simulink model "bicycle_car_model"  (R2019b)
settings: Solver=ode45  StartTime=0.0  StopTime=tf  MaxStep=0.01  RelTol=1e-3
undefined symbols (not defined in the file): a, accel_noise, accel_ts, b, Cf, Cr_MR, Cr_R, d0, gyro_noise, gyro_ts, initial, Jy, Ku_MR, Ku_R, m, mag_noise, mag_ts, mu, Nf, Nr, sf, sr, ti, U
libraries: simulink x5
settings Model: Creator=lclemen  LastModifiedBy=lclemen

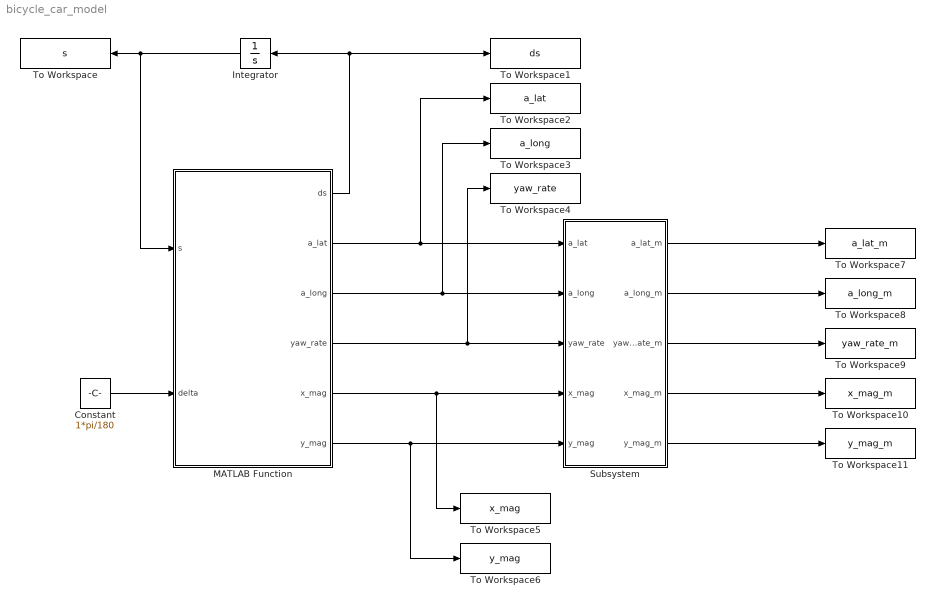
== system bicycle_car_model ==
  Constant : Constant  Value=1*pi/180
  Integrator : Integrator  InitialCondition=initial
  MATLAB Function : MATLAB Function  TreatAsAtomicUnit=on
  Subsystem : Subsystem
  To Workspace : ToWorkspace  VariableName=s  SampleTime=-1
      settings: Save2DSignal=2-D array (concatenate along first dimension)
  To Workspace1 : ToWorkspace  VariableName=ds  SampleTime=-1
      settings: Save2DSignal=2-D array (concatenate along first dimension)
  To Workspace10 : ToWorkspace  VariableName=x_mag_m  SampleTime=-1
      settings: Save2DSignal=2-D array (concatenate along first dimension)
  To Workspace11 : ToWorkspace  VariableName=y_mag_m  SampleTime=-1
      settings: Save2DSignal=2-D array (concatenate along first dimension)
  To Workspace2 : ToWorkspace  VariableName=a_lat  SampleTime=-1
      settings: Save2DSignal=2-D array (concatenate along first dimension)
  To Workspace3 : ToWorkspace  VariableName=a_long  SampleTime=-1
      settings: Save2DSignal=2-D array (concatenate along first dimension)
  To Workspace4 : ToWorkspace  VariableName=yaw_rate  SampleTime=-1
      settings: Save2DSignal=2-D array (concatenate along first dimension)
  To Workspace5 : ToWorkspace  VariableName=x_mag  SampleTime=-1
      settings: Save2DSignal=2-D array (concatenate along first dimension)
  To Workspace6 : ToWorkspace  VariableName=y_mag  SampleTime=-1
      settings: Save2DSignal=2-D array (concatenate along first dimension)
  To Workspace7 : ToWorkspace  VariableName=a_lat_m  SampleTime=-1
      settings: Save2DSignal=2-D array (concatenate along first dimension)
  To Workspace8 : ToWorkspace  VariableName=a_long_m  SampleTime=-1
      settings: Save2DSignal=2-D array (concatenate along first dimension)
  To Workspace9 : ToWorkspace  VariableName=yaw_rate_m  SampleTime=-1
      settings: Save2DSignal=2-D array (concatenate along first dimension)
  wires:
  MATLAB Function/2(a_lat) -> Subsystem/1(a_lat), To Workspace2/1
  MATLAB Function/1(ds) -> Integrator/1, To Workspace1/1
  Integrator/1 -> To Workspace/1, MATLAB Function/1(s)
  Constant/1 -> MATLAB Function/2(delta)
  MATLAB Function/3(a_long) -> Subsystem/2(a_long), To Workspace3/1
  MATLAB Function/4(yaw_rate) -> Subsystem/3(yaw_rate), To Workspace4/1
  MATLAB Function/6(y_mag) -> To Workspace6/1, Subsystem/5(y_mag)
  MATLAB Function/5(x_mag) -> To Workspace5/1, Subsystem/4(x_mag)
  Subsystem/1(a_lat_m) -> To Workspace7/1
  Subsystem/2(a_long_m) -> To Workspace8/1
  Subsystem/3(yaw_rate_m) -> To Workspace9/1
  Subsystem/4(x_mag_m) -> To Workspace10/1
  Subsystem/5(y_mag_m) -> To Workspace11/1

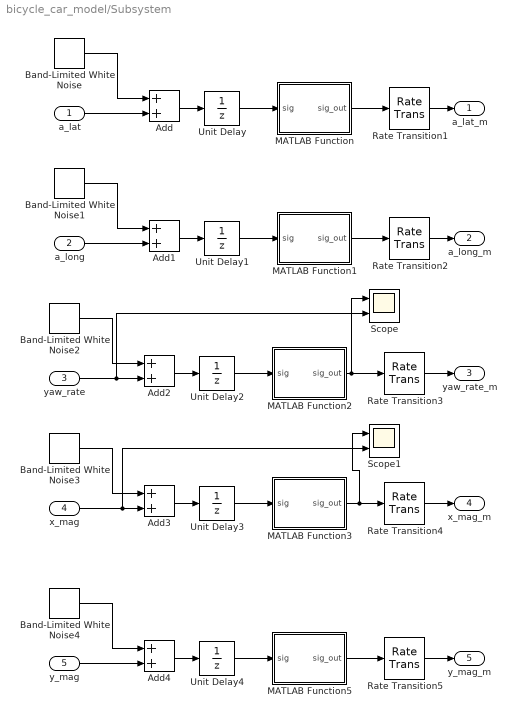
== system bicycle_car_model/Subsystem ==
  a_lat : Inport
  a_long : Inport  Port=2
  yaw_rate : Inport  Port=3
  x_mag : Inport  Port=4
  y_mag : Inport  Port=5
  Add{,1..4} (5 alike) : Sum
  Band-Limited White Noise : simulink/Sources/Band-Limited White Noise  Cov=[accel_noise]  Ts=0.001  seed=[23341]
  Band-Limited White Noise1 : simulink/Sources/Band-Limited White Noise  Cov=[accel_noise]  Ts=0.001  seed=[23341]
  Band-Limited White Noise2 : simulink/Sources/Band-Limited White Noise  Cov=[gyro_noise]  Ts=0.001  seed=[23341]
  Band-Limited White Noise3 : simulink/Sources/Band-Limited White Noise  Cov=[mag_noise]  Ts=0.001  seed=[23341]
  Band-Limited White Noise4 : simulink/Sources/Band-Limited White Noise  Cov=[accel_noise]  Ts=0.001  seed=[23341]
  MATLAB Function : MATLAB Function  TreatAsAtomicUnit=on
  MATLAB Function1 : MATLAB Function  TreatAsAtomicUnit=on
  MATLAB Function2 : MATLAB Function  TreatAsAtomicUnit=on
  MATLAB Function3 : MATLAB Function  TreatAsAtomicUnit=on
  MATLAB Function5 : MATLAB Function  TreatAsAtomicUnit=on
  Rate Transition{1..5} (5 alike) : RateTransition
  Scope : Scope  NumInputPorts=2
  Scope1 : Scope  NumInputPorts=2
  Unit Delay : UnitDelay  SampleTime=accel_ts  HasFrameUpgradeWarning=on
  Unit Delay1 : UnitDelay  SampleTime=accel_ts  HasFrameUpgradeWarning=on
  Unit Delay2 : UnitDelay  SampleTime=gyro_ts  HasFrameUpgradeWarning=on
  Unit Delay3 : UnitDelay  SampleTime=mag_ts  HasFrameUpgradeWarning=on
  Unit Delay4 : UnitDelay  SampleTime=accel_ts  HasFrameUpgradeWarning=on
  a_lat_m : Outport
  a_long_m : Outport  Port=2
  yaw_rate_m : Outport  Port=3
  x_mag_m : Outport  Port=4
  y_mag_m : Outport  Port=5
  wires:
  Band-Limited White Noise/1 -> Add/1
  a_lat/1 -> Add/2
  Add/1 -> Unit Delay/1
  Rate Transition1/1 -> a_lat_m/1
  Unit Delay/1 -> MATLAB Function/1(sig)
  MATLAB Function/1(sig_out) -> Rate Transition1/1
  Band-Limited White Noise1/1 -> Add1/1
  MATLAB Function1/1(sig_out) -> Rate Transition2/1
  Add1/1 -> Unit Delay1/1
  a_long/1 -> Add1/2
  Unit Delay1/1 -> MATLAB Function1/1(sig)
  Rate Transition2/1 -> a_long_m/1
  MATLAB Function2/1(sig_out) -> Scope/1, Rate Transition3/1
  Add2/1 -> Unit Delay2/1
  yaw_rate/1 -> Scope/2, Add2/2
  Unit Delay2/1 -> MATLAB Function2/1(sig)
  Band-Limited White Noise2/1 -> Add2/1
  Rate Transition3/1 -> yaw_rate_m/1
  MATLAB Function3/1(sig_out) -> Scope1/1, Rate Transition4/1
  Add3/1 -> Unit Delay3/1
  x_mag/1 -> Scope1/2, Add3/2
  Unit Delay3/1 -> MATLAB Function3/1(sig)
  Band-Limited White Noise3/1 -> Add3/1
  Rate Transition4/1 -> x_mag_m/1
  MATLAB Function5/1(sig_out) -> Rate Transition5/1
  Add4/1 -> Unit Delay4/1
  y_mag/1 -> Add4/2
  Unit Delay4/1 -> MATLAB Function5/1(sig)
  Band-Limited White Noise4/1 -> Add4/1
  Rate Transition5/1 -> y_mag_m/1

== matlab function bicycle_car_model/Subsystem/MATLAB Function ==
  data: sig input; sig_out output; accel_res parameter
function sig_out = accel_quant(sig, accel_res)
% based on 16-bit signal with +/- 4g
sig_out = round(sig/accel_res)*accel_res;

== matlab function bicycle_car_model/MATLAB Function ==
  data: s input; delta input; ds output; a_lat output; m parameter; b parameter; a parameter; Cf parameter; Jy parameter; U parameter; Ku_MR parameter; Cr_MR parameter; mu parameter; Ku_R parameter; Cr_R parameter; sf parameter; sr parameter; Nf parameter; Nr parameter; ti parameter; d0 parameter; a_long output; yaw_rate output; x_mag output; y_mag output
%% Equations file for simulation 2 - Planar handling model.  
function [ds, a_lat, a_long, yaw_rate, x_mag, y_mag] = eqns(s, delta, m, b, a, Cf, Jy, U, Ku_MR, Cr_MR, mu, Ku_R, Cr_R, sf, sr, Nf, Nr, ti, d0)


%% Variable initialization - omega = theta_dot
% Reference car
V = s(1);
theta = s(2);
omega = s(3);
x = s(4);
y = s(5);


ds = zeros(5,1);
ext = zeros(10,1);

%% Inputs
% Delta
% if t > ti
%     delta = d0*pi/180;
% else 
%     delta = 0;
% end
% 
% delta = d0*pi/180*sin(2*pi*t);

%% Gain schedule for Ki and Kp
% This was found using the MATLAB PID tuning tool. The final equations were
% found by tuning the gains for a settling time of magnitude 10^-2 and then
% assuming that the gains for change from the found Ts to a Ts of 0.02 were 
% proportional. These were then curve fit in Excel. 
Ki = 0.5*1903*U^(-0.916);
Kp = 0.5*(0.0556*U + 6.0513);

%% Calculation of side force - Reference Car
% alpha = wheel slip angle and F = Ca*alpha
alpha_f = delta - (V + a*omega)/U;
alpha_r = (b*omega-V)/U;
Ff = Cf*alpha_f;
Fr = Cr_MR*alpha_r;

%% Calculation of side force - Real Car
% alpha = wheel slip angle and F = Ca*alpha
% err = omega-omega_R;
% delta_c = Kp*err + Ki*erri;
% alpha_f_R = delta_c - (V_R + a*omega_R)/U;
% alpha_r_R = (b*omega_R-V_R)/U;

% %For the front
% F_xd_f=Cf*sf/(1-sf);
% F_yd_f=Cf*tan(alpha_f_R)/(1-sf);
% Q_f=sqrt( (F_xd_f/Nf)^2+(F_yd_f/Nf)^2 );
% if Q_f==0;
%     Q_f=.0001;                       %Makes sure there is no divide by zero
% end;
% lambda_f=mu/2/Q_f;
% if lambda_f >=1;
%     Fx_f=F_xd_f; Fy_f=F_yd_f;
% else
%    Fx_f=F_xd_f*2*lambda_f*(1-lambda_f/2);
%    Fy_f=F_yd_f*2*lambda_f*(1-lambda_f/2);
% end;
% Ff_R=Fy_f;
% 
% %For the rear
% F_xd_r=Cr_R*sr/(1-sr);
% F_yd_r=Cr_R*tan(alpha_r_R)/(1-sr);
% Q_r=sqrt((F_xd_r/Nr)^2+(F_yd_r/Nr)^2 );
% if Q_r == 0;
%     Q_r=.0001;                    %Makes sure there is no divide by zero
% end;
% lambda_r=mu/2/Q_r;
% if lambda_r >=1;
%     Fx_r=F_xd_r; Fy_r=F_yd_r;
% else
%    Fx_r=F_xd_r*2*lambda_r*(1-lambda_r/2);
%    Fy_r=F_yd_r*2*lambda_r*(1-lambda_r/2);
% end;
% Fr_R=Fy_r;

%% Equations of Motion - Reference Car
V_dot = Ff/m + Fr/m - U*omega;
theta_dot = omega;
omega_dot = a*Ff/Jy - b*Fr/Jy;
x_dot = U*cos(theta) - V*sin(theta);
y_dot = U*sin(theta) + V*cos(theta);

% %% Equations of Motion - Real Car
% V_dot_R = Ff_R/m + Fr_R/m - U*omega_R;
% theta_dot_R = omega_R;
% omega_dot_R = a*Ff_R/Jy - b*Fr_R/Jy;
% x_dot_R = U*cos(theta_R) - V_R*sin(theta_R);
% y_dot_R = U*sin(theta_R) + V_R*cos(theta_R);
% erri_dot = err;

%% Extra outputs
a_lat = Ff/m + Fr/m;
a_long = Ff*sin(delta)/m;
yaw_rate = omega;
x_mag = 4900*cos(theta);
y_mag = 4900*sin(theta);
% ext(1) = Ff;
% ext(2) = Fr;
% ext(3) = alpha_f;
% ext(4) = alpha_r;
% ext(5) = delta;

ds = [V_dot; theta_dot; omega_dot; x_dot; y_dot];

== matlab function bicycle_car_model/Subsystem/MATLAB Function1 ==
  data: sig input; sig_out output; accel_res parameter
function sig_out = accel_quant(sig, accel_res)
% based on 16-bit signal with +/- 4g
sig_out = round(sig/accel_res)*accel_res;

== matlab function bicycle_car_model/Subsystem/MATLAB Function2 ==
  data: sig input; sig_out output; gyro_res parameter
function sig_out = gyro_quant(sig, gyro_res)
% based on 16-bit signal with +/- 4g
sig_out = round(sig/gyro_res)*gyro_res;

== matlab function bicycle_car_model/Subsystem/MATLAB Function3 ==
  data: sig input; sig_out output; mag_res parameter
function sig_out = mag_quant(sig, mag_res)
% based on 16-bit signal with +/- 4g
sig_out = round(sig/mag_res)*mag_res;

== matlab function bicycle_car_model/Subsystem/MATLAB Function5 ==
  data: sig input; sig_out output; mag_res parameter
function sig_out = mag_quant(sig, mag_res)
% based on 16-bit signal with +/- 4g
sig_out = round(sig/mag_res)*mag_res;
